simulink model "RLC_ex9"  (R2021b)
settings: Solver=VariableStepAuto  StartTime=0.0  StopTime=10.0  RelTol=1e-3
values from neighbouring files (symbols this model uses):
  C = 10e-6    (= 1e-05)    [ex10.m]    (also in ex27.m; ex27c.m = 1.05e-05; ex34.m = [B(2) B(4);c1 c2]; ex8.m)
  L = 1e-3    (= 0.001)    [ex10.m]    (also in ex23.m = 0.2; ex27.m = 0.0001; ex27c.m = 0.0001; ex8.m)
  R = Rv(n)    [ex10.m]    (also in ex22.m = 0.2; ex23.m = 1.3; ex27c.m = 2.8; ex8.m = 10)
settings Model: Creator=rafam  LastModifiedBy=rafam

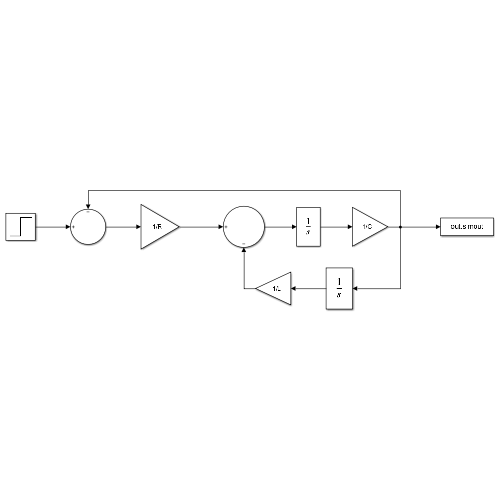
[thumbnail: Simulink's stored preview of the top-level diagram]
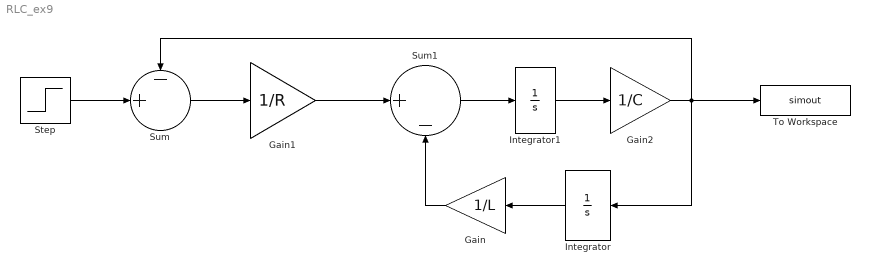
== system RLC_ex9 ==
  Gain : Gain  Gain=1/L
  Gain1 : Gain  Gain=1/R
  Gain2 : Gain  Gain=1/C
  Integrator : Integrator
  Integrator1 : Integrator
  Step : Step  Time=0  After=2  SampleTime=0
  Sum : Sum  Inputs=-+|
  Sum1 : Sum  Inputs=|+-
  To Workspace : ToWorkspace  VariableName=simout  SaveFormat=Timeseries  SampleTime=-1
  wires:
  Sum/1 -> Gain1/1
  Gain1/1 -> Sum1/1
  Sum1/1 -> Integrator1/1
  Integrator1/1 -> Gain2/1
  Integrator/1 -> Gain/1
  Gain/1 -> Sum1/2
  Gain2/1 -> Sum/1, To Workspace/1, Integrator/1
  Step/1 -> Sum/2
